simulink model "msdft_12_v2"  (R2013b)
settings: Solver=ode45  StartTime=0.0  StopTime=10.0  RelTol=1e-3
undefined symbols (not defined in the file or in its folder): msdft, sys_lib
libraries: xbsIndex_r4 x3195, casper_library_misc x152, casper_library_delays x42, dspsigops x32, xps_library x3
(part 10 of 33)

== system msdft_12_v2/msdft1/delay_tree4 ==
  in : Inport
  delay_c1_r1 : xbsIndex_r4/Delay  rst=off  infoeditControl=Selection of Reset will increase slice count due to use of real FFs and instead of SRLs  en=off  latency=1  dbl_ovrd=off  reg_retiming=on  block_type=delay
      settings: block_version=11.4
  delay_c2_r1 : xbsIndex_r4/Delay  rst=off  infoeditControl=Selection of Reset will increase slice count due to use of real FFs and instead of SRLs  en=off  latency=1  dbl_ovrd=off  reg_retiming=on  block_type=delay
      settings: block_version=11.4
  delay_c2_r2 : xbsIndex_r4/Delay  rst=off  infoeditControl=Selection of Reset will increase slice count due to use of real FFs and instead of SRLs  en=off  latency=1  dbl_ovrd=off  reg_retiming=on  block_type=delay
      settings: block_version=11.4
  delay_c3_r{1..4} (4 alike) : xbsIndex_r4/Delay  rst=off  infoeditControl=Selection of Reset will increase slice count due to use of real FFs and instead of SRLs  en=off  latency=1  dbl_ovrd=off  reg_retiming=on  block_type=delay
  delay_c4_r{1..8} (8 alike) : xbsIndex_r4/Delay  rst=off  infoeditControl=Selection of Reset will increase slice count due to use of real FFs and instead of SRLs  en=off  latency=1  dbl_ovrd=off  reg_retiming=on  block_type=delay
  term6 : Terminator
  term7 : Terminator
  term8 : Terminator
  out1 : Outport
  out2 : Outport  Port=2
  out3 : Outport  Port=3
  out4 : Outport  Port=4
  out5 : Outport  Port=5
  wires:
  in/1 -> delay_c1_r1/1
  delay_c1_r1/1 -> delay_c2_r1/1, delay_c2_r2/1
  delay_c2_r1/1 -> delay_c3_r1/1, delay_c3_r2/1
  delay_c2_r2/1 -> delay_c3_r3/1, delay_c3_r4/1
  delay_c3_r1/1 -> delay_c4_r1/1, delay_c4_r2/1
  delay_c3_r2/1 -> delay_c4_r3/1, delay_c4_r4/1
  delay_c3_r3/1 -> delay_c4_r5/1, delay_c4_r6/1
  delay_c3_r4/1 -> delay_c4_r7/1, delay_c4_r8/1
  delay_c4_r1/1 -> out1/1
  delay_c4_r2/1 -> out2/1
  delay_c4_r3/1 -> out3/1
  delay_c4_r4/1 -> out4/1
  delay_c4_r5/1 -> out5/1
  delay_c4_r6/1 -> term6/1
  delay_c4_r7/1 -> term7/1
  delay_c4_r8/1 -> term8/1

== system msdft_12_v2/msdft1/delay_tree5 ==
  in : Inport
  delay_c1_r1 : xbsIndex_r4/Delay  rst=off  infoeditControl=Selection of Reset will increase slice count due to use of real FFs and instead of SRLs  en=off  latency=1  dbl_ovrd=off  reg_retiming=on  block_type=delay
      settings: block_version=11.4
  delay_c2_r1 : xbsIndex_r4/Delay  rst=off  infoeditControl=Selection of Reset will increase slice count due to use of real FFs and instead of SRLs  en=off  latency=1  dbl_ovrd=off  reg_retiming=on  block_type=delay
      settings: block_version=11.4
  delay_c2_r2 : xbsIndex_r4/Delay  rst=off  infoeditControl=Selection of Reset will increase slice count due to use of real FFs and instead of SRLs  en=off  latency=1  dbl_ovrd=off  reg_retiming=on  block_type=delay
      settings: block_version=11.4
  delay_c3_r{1..4} (4 alike) : xbsIndex_r4/Delay  rst=off  infoeditControl=Selection of Reset will increase slice count due to use of real FFs and instead of SRLs  en=off  latency=1  dbl_ovrd=off  reg_retiming=on  block_type=delay
  delay_c4_r{1..8} (8 alike) : xbsIndex_r4/Delay  rst=off  infoeditControl=Selection of Reset will increase slice count due to use of real FFs and instead of SRLs  en=off  latency=1  dbl_ovrd=off  reg_retiming=on  block_type=delay
  term6 : Terminator
  term7 : Terminator
  term8 : Terminator
  out1 : Outport
  out2 : Outport  Port=2
  out3 : Outport  Port=3
  out4 : Outport  Port=4
  out5 : Outport  Port=5
  wires:
  in/1 -> delay_c1_r1/1
  delay_c1_r1/1 -> delay_c2_r1/1, delay_c2_r2/1
  delay_c2_r1/1 -> delay_c3_r1/1, delay_c3_r2/1
  delay_c2_r2/1 -> delay_c3_r3/1, delay_c3_r4/1
  delay_c3_r1/1 -> delay_c4_r1/1, delay_c4_r2/1
  delay_c3_r2/1 -> delay_c4_r3/1, delay_c4_r4/1
  delay_c3_r3/1 -> delay_c4_r5/1, delay_c4_r6/1
  delay_c3_r4/1 -> delay_c4_r7/1, delay_c4_r8/1
  delay_c4_r1/1 -> out1/1
  delay_c4_r2/1 -> out2/1
  delay_c4_r3/1 -> out3/1
  delay_c4_r4/1 -> out4/1
  delay_c4_r5/1 -> out5/1
  delay_c4_r6/1 -> term6/1
  delay_c4_r7/1 -> term7/1
  delay_c4_r8/1 -> term8/1

== system msdft_12_v2/msdft1/delay_tree6 ==
  in : Inport
  delay_c1_r1 : xbsIndex_r4/Delay  rst=off  infoeditControl=Selection of Reset will increase slice count due to use of real FFs and instead of SRLs  en=off  latency=1  dbl_ovrd=off  reg_retiming=on  block_type=delay
      settings: block_version=11.4
  delay_c2_r1 : xbsIndex_r4/Delay  rst=off  infoeditControl=Selection of Reset will increase slice count due to use of real FFs and instead of SRLs  en=off  latency=1  dbl_ovrd=off  reg_retiming=on  block_type=delay
      settings: block_version=11.4
  delay_c2_r2 : xbsIndex_r4/Delay  rst=off  infoeditControl=Selection of Reset will increase slice count due to use of real FFs and instead of SRLs  en=off  latency=1  dbl_ovrd=off  reg_retiming=on  block_type=delay
      settings: block_version=11.4
  delay_c3_r{1..4} (4 alike) : xbsIndex_r4/Delay  rst=off  infoeditControl=Selection of Reset will increase slice count due to use of real FFs and instead of SRLs  en=off  latency=1  dbl_ovrd=off  reg_retiming=on  block_type=delay
  delay_c4_r{1..8} (8 alike) : xbsIndex_r4/Delay  rst=off  infoeditControl=Selection of Reset will increase slice count due to use of real FFs and instead of SRLs  en=off  latency=1  dbl_ovrd=off  reg_retiming=on  block_type=delay
  term6 : Terminator
  term7 : Terminator
  term8 : Terminator
  out1 : Outport
  out2 : Outport  Port=2
  out3 : Outport  Port=3
  out4 : Outport  Port=4
  out5 : Outport  Port=5
  wires:
  in/1 -> delay_c1_r1/1
  delay_c1_r1/1 -> delay_c2_r1/1, delay_c2_r2/1
  delay_c2_r1/1 -> delay_c3_r1/1, delay_c3_r2/1
  delay_c2_r2/1 -> delay_c3_r3/1, delay_c3_r4/1
  delay_c3_r1/1 -> delay_c4_r1/1, delay_c4_r2/1
  delay_c3_r2/1 -> delay_c4_r3/1, delay_c4_r4/1
  delay_c3_r3/1 -> delay_c4_r5/1, delay_c4_r6/1
  delay_c3_r4/1 -> delay_c4_r7/1, delay_c4_r8/1
  delay_c4_r1/1 -> out1/1
  delay_c4_r2/1 -> out2/1
  delay_c4_r3/1 -> out3/1
  delay_c4_r4/1 -> out4/1
  delay_c4_r5/1 -> out5/1
  delay_c4_r6/1 -> term6/1
  delay_c4_r7/1 -> term7/1
  delay_c4_r8/1 -> term8/1

== system msdft_12_v2/msdft1/msdft ==
  note: see if saturates
  note: zero before
      | sync
  din : Inport
  sync : Inport  Port=2
  rst : Inport  Port=3
  twidd_im : Inport  Port=4
  twidd_re : Inport  Port=5
  we_twidd : Inport  Port=6
  mem_addr : Inport  Port=7
  Constant : xbsIndex_r4/Constant  const=1  gui_display_data_type=Boolean  arith_type=Boolean  n_bits=16  bin_pt=14  preci_type=Single  exp_width=8  frac_width=24  explicit_period=on  period=1  equ=P=C  opselect=C  inp2=PCIN>>17  opr=+  inp1=P  carry=CIN  dbl_ovrd=off  block_type=constant
  Convert : xbsIndex_r4/Convert  gui_display_data_type=Fixed-point  arith_type="Signed  (2's comp)"  n_bits=32  bin_pt=30  float_type=Single  exp_bits=8  fraction_bits=24  quantization=Truncate  overflow=Wrap  en=off  latency=0  dbl_ovrd=off  pipeline=off  block_type=convert
      settings: block_version=11.4
  Convert1 : xbsIndex_r4/Convert  gui_display_data_type=Fixed-point  arith_type="Signed  (2's comp)"  n_bits=32  bin_pt=30  float_type=Single  exp_bits=8  fraction_bits=24  quantization=Truncate  overflow=Wrap  en=off  latency=0  dbl_ovrd=off  pipeline=off  block_type=convert
      settings: block_version=11.4
  Delay : xbsIndex_r4/Delay  rst=off  infoeditControl=Selection of Reset will increase slice count due to use of real FFs and instead of SRLs  en=off  latency=5  dbl_ovrd=off  reg_retiming=off  block_type=delay
  Reinterpret : xbsIndex_r4/Reinterpret  force_arith_type=off  arith_type=Unsigned  force_bin_pt=on  bin_pt=twidd_bit-2  block_type=reinterpret
  Reinterpret1 : xbsIndex_r4/Reinterpret  force_arith_type=off  arith_type=Unsigned  force_bin_pt=on  bin_pt=twidd_bit-2  block_type=reinterpret
  Terminator : Terminator
  c_to_ri : casper_library_misc/c_to_ri  n_bits=16  bin_pt=14
      settings: AttributesFormatString=16_14 r/i
  cmult : Subsystem  AncestorBlock=casper_library_multipliers/cmult  mask(cmult){n_bits_a=in_bit+1, bin_pt_a=in_bit-1, n_bits_b=twidd_bit, bin_pt_b=twidd_bit-2, n_bits_ab=out_bit-N, bin_pt_ab=out_bit-N-5, quantization=Round  (unbiased: Even Values), overflow=Wrap, in_latency=0, mult_latency=3, add_latency=1, conv_latency=1, conjugated=off, async=off, pipelined_enable=on, multiplier_implementation=behavioral HDL}
      mask prompts: n_bits_a "Number of Bits 'a'"; bin_pt_a "Binary Point 'a'"; n_bits_b "Number of Bits 'b'"; bin_pt_b "Binary Point 'b'"; n_bits_ab "Number of Bits 'ab'"; bin_pt_ab "Binary Point 'ab'"; in_latency "Input latency"; mult_latency "Multiplier Latency"; add_latency "Adder Latency"; conv_latency "Convert latency"; conjugated "Conjugate"; async "asynchronous operation"; pipelined_enable "enable pipeline"; multiplier_implementation "Multiplier implementation"
      mask help:
      | Multiplies two complex numbers using 4 multipliers and 2 adders.
      | Conjugation is optional.
      mask init: same as msdft_12_v2/corrs/Subsystem/cmult
      settings: AttributesFormatString=|
      | 9_7 * 16_14 ==> 13_8
      | Round  (unbiased: Even Values), Wrap
      | Latency=0
      mask TypeOptions quantization: Truncate | Round  (unbiased: +/- Inf) | Round  (unbiased: Even Values)
      mask TypeOptions overflow: Wrap | Saturate | Flag as error
      mask TypeOptions multiplier_implementation: behavioral HDL | standard core | embedded multiplier core
  comb_filter : Subsystem  mask{N=N, bitwidth=in_bit}
      mask prompts: N "fft length (2^N)"
  done : Subsystem  Tag=xps:sw_reg  AncestorBlock=xps_library/software_register  mask(swreg){io_dir=To Processor, io_delay=0, sample_period=1, names=reg, bitwidths=32, bin_pts=0, arith_types=2, sim_port=on, show_format=on}
      mask prompts: io_dir "I/O direction"; io_delay "I/O delay"; sample_period "Sample period"; names "Bitfield names [msb...lsb]"; bitwidths "Bitfield widths"; bin_pts "Bitfield binary pts"; arith_types "Bitfield types, ufix=0, fix=1, bool=2"; sim_port "Provide sim input/output?"; show_format "Print format string?"
      mask help: A 32-bit software-accessible register. Can be divided into bitfields of varying widths and types using the fields in the block mask.
      mask init:
      | try
      |     swreg_init(gcb)
      | catch ex
      |     disp(sprintf('%s: %s', gcb, ex.message))
      |     errordlg(ex.message)
      | end
      settings: AttributesFormatString=1output:b = 32 bits
      mask TypeOptions io_dir: To Processor | From Processor
      mask Callback io_dir:
      | mask_enables = get_param(gcb, 'MaskEnables');
      | mask_names = get_param(gcb, 'MaskNames');
      | if strcmp(get_param(gcb, 'io_dir'), 'To Processor'),
      |     mask_enables{ismember(mask_names, 'sample_period')} = 'off';
      | else
      |     mask_enables{ismember(mask_names, 'sample_period')} = 'on';
      | end
      | set_param(gcb, 'MaskEnables', mask_enables);
  freeze_cntr : casper_library_misc/freeze_cntr  CounterBits=12
  pulse_ext : casper_library_misc/pulse_ext  pulse_len=2^8
  resonator : Subsystem  mask{in_bitwidth=out_bit-N, in_point=out_bit-N-5, N=N}
      mask prompts: in_bitwidth "input bitwidth"; in_point "input point"; N "fft length (2^?)"
  ri_to_c : casper_library_misc/ri_to_c
  rst_bram : Subsystem  Tag=xps:sw_reg  AncestorBlock=xps_library/software_register  mask(swreg){io_dir=From Processor, io_delay=0, sample_period=1, names=reg, bitwidths=32, bin_pts=0, arith_types=2, sim_port=on, show_format=on}
      mask prompts: io_dir "I/O direction"; io_delay "I/O delay"; sample_period "Sample period"; names "Bitfield names [msb...lsb]"; bitwidths "Bitfield widths"; bin_pts "Bitfield binary pts"; arith_types "Bitfield types, ufix=0, fix=1, bool=2"; sim_port "Provide sim input/output?"; show_format "Print format string?"
      mask help: A 32-bit software-accessible register. Can be divided into bitfields of varying widths and types using the fields in the block mask.
      mask init:
      | try
      |     swreg_init(gcb)
      | catch ex
      |     disp(sprintf('%s: %s', gcb, ex.message))
      |     errordlg(ex.message)
      | end
      settings: AttributesFormatString=1input:b = 32 bits
      mask TypeOptions io_dir: To Processor | From Processor
      mask Callback io_dir:
      | mask_enables = get_param(gcb, 'MaskEnables');
      | mask_names = get_param(gcb, 'MaskNames');
      | if strcmp(get_param(gcb, 'io_dir'), 'To Processor'),
      |     mask_enables{ismember(mask_names, 'sample_period')} = 'off';
      | else
      |     mask_enables{ismember(mask_names, 'sample_period')} = 'on';
      | end
      | set_param(gcb, 'MaskEnables', mask_enables);
  snapshot : Subsystem  Tag=casper:snapshot  AncestorBlock=casper_library_scopes/snapshot  mask(snapshot){storage=bram, dram_dimm=1, dram_clock=200, nsamples=10, data_width=64, offset=off, circap=off, value=off, use_dsp48=on}
      mask prompts: storage "Storage medium"; dram_dimm "DRAM dimm"; dram_clock "DRAM clock rate"; nsamples "Number of Samples (2^?)"; data_width "Data width"; offset "Start delay support"; circap "Circular capture support"; value "Extra value capture support"; use_dsp48 "Use DSP48s to implement counters"
      mask help:
      | Standard snap block, but with the following optional extras;
      |  1) Optionally delay the fabric trigger by a user-specified number of valids.
      |  2) Capture continuously after a trigger until a stop pulse is received. Data is captured into BRAM continuously, with old data being overwritten until a stop command is received. Then stop capturing when memory is filled. This enables you to get some data before and some data after the stop pulse. Use the 'tr_en_cnt' register to determine where you are in your vector. 'Addr' register's MSb now indicates 'busy capturing'.
      |  3) Optionally capture a value on an input port to a register at the same time as the first data sample.
      |  4) Implement counters using DSP48Es to save resources.
      mask init: same as msdft_12_v2/snapshot
      mask TypeOptions storage: bram | dram
      mask Callback storage: snapshot_callback();
      mask TypeOptions dram_dimm: 1 | 2 | 3 | 4
      mask TypeOptions dram_clock: 200 | 250 | 266 | 300 | 333
      mask TypeOptions data_width: 8 | 16 | 32 | 64 | 128
  twiddle_factor : Subsystem  mask{N=N, k=init_twidd, bitsize=twidd_bit}
      mask prompts: N "length FFT(2^)"; k "twiddle factor"; bitsize "bit size"
      mask help: RAM memories containing the twiddle adequate twiddle factors
  twidds : Subsystem  Tag=xps:bram  AncestorBlock=xps_library/Shared_BRAM  mask{arith_type=Unsigned, addr_width=12, data_width=64, reg_prim_output=off, reg_core_output=off, optimization=Minimum_Area, data_bin_pt=0, init_vals=[0:2^10-1], sample_rate=1}
      mask prompts: arith_type "Output Data Type"; addr_width "Address width"; data_width "Data Width"; reg_prim_output "Register Primitive Output"; reg_core_output "Register Core Output"; data_bin_pt "Data Binary Point"; init_vals "Initial values (simulation only)"; sample_rate "Sample rate"
      mask init:
      | shared_bram_mask;
      mask TypeOptions arith_type: Unsigned | Signed  (2's comp)
      mask TypeOptions data_width: 8 | 16 | 32 | 64 | 128
      mask TypeOptions optimization: Minimum_Area | Low_Power
  dout : Outport
  wires:
  Reinterpret1/1 -> twiddle_factor/6(im_data)
  Reinterpret/1 -> twiddle_factor/5(re_data)
  we_twidd/1 -> twiddle_factor/4(we_mem)
  sync/1 -> comb_filter/3(sync)
  [rst] -> comb_filter/2(rst)
  rst/1 -> [rst]
  comb_filter/1(dout) -> cmult/1(a)
  [rst] -> resonator/3(rst)
  Delay/1 -> resonator/2(sync)
  cmult/1(ab) -> resonator/1(din)
  twiddle_factor/2(sync_out) -> pulse_ext/1, Delay/1
  twiddle_factor/1(dout) -> cmult/2(b), c_to_ri/1
  twidd_im/1 -> Reinterpret1/1
  twidd_re/1 -> Reinterpret/1
  mem_addr/1 -> twiddle_factor/3(dir_mem)
  [rst] -> twiddle_factor/1(rst)
  comb_filter/2(sync_out) -> twiddle_factor/2(sync)
  resonator/1(dout) -> dout/1
  din/1 -> comb_filter/1(din)
  c_to_ri/1 -> Convert/1
  c_to_ri/2 -> Convert1/1
  Convert/1 -> ri_to_c/1
  Convert1/1 -> ri_to_c/2
  freeze_cntr/2 -> twidds/3(we)
  ri_to_c/1 -> snapshot/1(din), twidds/2(data_in)
  freeze_cntr/1 -> twidds/1(addr)
  pulse_ext/1 -> freeze_cntr/1
  rst_bram/1(in_reg) -> freeze_cntr/2
  freeze_cntr/3 -> done/1(out_reg)
  twidds/1(data_out) -> Terminator/1
  Constant/1 -> snapshot/2(we), snapshot/3(trig)

== system msdft_12_v2/msdft1/msdft1 ==
  note: see if saturates
  note: zero before
      | sync
  din : Inport
  sync : Inport  Port=2
  rst : Inport  Port=3
  twidd_im : Inport  Port=4
  twidd_re : Inport  Port=5
  we_twidd : Inport  Port=6
  mem_addr : Inport  Port=7
  Delay : xbsIndex_r4/Delay  rst=off  infoeditControl=Selection of Reset will increase slice count due to use of real FFs and instead of SRLs  en=off  latency=5  dbl_ovrd=off  reg_retiming=off  block_type=delay
  Reinterpret : xbsIndex_r4/Reinterpret  force_arith_type=off  arith_type=Unsigned  force_bin_pt=on  bin_pt=twidd_bit-2  block_type=reinterpret
  Reinterpret1 : xbsIndex_r4/Reinterpret  force_arith_type=off  arith_type=Unsigned  force_bin_pt=on  bin_pt=twidd_bit-2  block_type=reinterpret
  cmult : Subsystem  AncestorBlock=casper_library_multipliers/cmult  mask(cmult){n_bits_a=in_bit+1, bin_pt_a=in_bit-1, n_bits_b=twidd_bit, bin_pt_b=twidd_bit-2, n_bits_ab=out_bit-N, bin_pt_ab=out_bit-N-5, quantization=Round  (unbiased: Even Values), overflow=Wrap, in_latency=0, mult_latency=3, add_latency=1, conv_latency=1, conjugated=off, async=off, pipelined_enable=on, multiplier_implementation=behavioral HDL}
      mask prompts: n_bits_a "Number of Bits 'a'"; bin_pt_a "Binary Point 'a'"; n_bits_b "Number of Bits 'b'"; bin_pt_b "Binary Point 'b'"; n_bits_ab "Number of Bits 'ab'"; bin_pt_ab "Binary Point 'ab'"; in_latency "Input latency"; mult_latency "Multiplier Latency"; add_latency "Adder Latency"; conv_latency "Convert latency"; conjugated "Conjugate"; async "asynchronous operation"; pipelined_enable "enable pipeline"; multiplier_implementation "Multiplier implementation"
      mask help:
      | Multiplies two complex numbers using 4 multipliers and 2 adders.
      | Conjugation is optional.
      mask init: same as msdft_12_v2/corrs/Subsystem/cmult
      settings: AttributesFormatString=|
      | 9_7 * 16_14 ==> 13_8
      | Round  (unbiased: Even Values), Wrap
      | Latency=0
      mask TypeOptions quantization: Truncate | Round  (unbiased: +/- Inf) | Round  (unbiased: Even Values)
      mask TypeOptions overflow: Wrap | Saturate | Flag as error
      mask TypeOptions multiplier_implementation: behavioral HDL | standard core | embedded multiplier core
  comb_filter : Subsystem  mask{N=N, bitwidth=in_bit}
      mask prompts: N "fft length (2^N)"
  resonator : Subsystem  mask{in_bitwidth=out_bit-N, in_point=out_bit-N-5, N=N}
      mask prompts: in_bitwidth "input bitwidth"; in_point "input point"; N "fft length (2^?)"
  twiddle_factor : Subsystem  mask{N=N, k=init_twidd, bitsize=twidd_bit}
      mask prompts: N "length FFT(2^)"; k "twiddle factor"; bitsize "bit size"
      mask help: RAM memories containing the twiddle adequate twiddle factors
  dout : Outport
  wires:
  Reinterpret1/1 -> twiddle_factor/6(im_data)
  Reinterpret/1 -> twiddle_factor/5(re_data)
  we_twidd/1 -> twiddle_factor/4(we_mem)
  sync/1 -> comb_filter/3(sync)
  [rst] -> comb_filter/2(rst)
  rst/1 -> [rst]
  comb_filter/1(dout) -> cmult/1(a)
  [rst] -> resonator/3(rst)
  Delay/1 -> resonator/2(sync)
  cmult/1(ab) -> resonator/1(din)
  twiddle_factor/2(sync_out) -> Delay/1
  twiddle_factor/1(dout) -> cmult/2(b)
  twidd_im/1 -> Reinterpret1/1
  twidd_re/1 -> Reinterpret/1
  mem_addr/1 -> twiddle_factor/3(dir_mem)
  [rst] -> twiddle_factor/1(rst)
  comb_filter/2(sync_out) -> twiddle_factor/2(sync)
  resonator/1(dout) -> dout/1
  din/1 -> comb_filter/1(din)

== system msdft_12_v2/msdft1/msdft2 ==
  note: see if saturates
  note: zero before
      | sync
  din : Inport
  sync : Inport  Port=2
  rst : Inport  Port=3
  twidd_im : Inport  Port=4
  twidd_re : Inport  Port=5
  we_twidd : Inport  Port=6
  mem_addr : Inport  Port=7
  Delay : xbsIndex_r4/Delay  rst=off  infoeditControl=Selection of Reset will increase slice count due to use of real FFs and instead of SRLs  en=off  latency=5  dbl_ovrd=off  reg_retiming=off  block_type=delay
  Reinterpret : xbsIndex_r4/Reinterpret  force_arith_type=off  arith_type=Unsigned  force_bin_pt=on  bin_pt=twidd_bit-2  block_type=reinterpret
  Reinterpret1 : xbsIndex_r4/Reinterpret  force_arith_type=off  arith_type=Unsigned  force_bin_pt=on  bin_pt=twidd_bit-2  block_type=reinterpret
  cmult : Subsystem  AncestorBlock=casper_library_multipliers/cmult  mask(cmult){n_bits_a=in_bit+1, bin_pt_a=in_bit-1, n_bits_b=twidd_bit, bin_pt_b=twidd_bit-2, n_bits_ab=out_bit-N, bin_pt_ab=out_bit-N-5, quantization=Round  (unbiased: Even Values), overflow=Wrap, in_latency=0, mult_latency=3, add_latency=1, conv_latency=1, conjugated=off, async=off, pipelined_enable=on, multiplier_implementation=behavioral HDL}
      mask prompts: n_bits_a "Number of Bits 'a'"; bin_pt_a "Binary Point 'a'"; n_bits_b "Number of Bits 'b'"; bin_pt_b "Binary Point 'b'"; n_bits_ab "Number of Bits 'ab'"; bin_pt_ab "Binary Point 'ab'"; in_latency "Input latency"; mult_latency "Multiplier Latency"; add_latency "Adder Latency"; conv_latency "Convert latency"; conjugated "Conjugate"; async "asynchronous operation"; pipelined_enable "enable pipeline"; multiplier_implementation "Multiplier implementation"
      mask help:
      | Multiplies two complex numbers using 4 multipliers and 2 adders.
      | Conjugation is optional.
      mask init: same as msdft_12_v2/corrs/Subsystem/cmult
      settings: AttributesFormatString=|
      | 9_7 * 16_14 ==> 13_8
      | Round  (unbiased: Even Values), Wrap
      | Latency=0
      mask TypeOptions quantization: Truncate | Round  (unbiased: +/- Inf) | Round  (unbiased: Even Values)
      mask TypeOptions overflow: Wrap | Saturate | Flag as error
      mask TypeOptions multiplier_implementation: behavioral HDL | standard core | embedded multiplier core
  comb_filter : Subsystem  mask{N=N, bitwidth=in_bit}
      mask prompts: N "fft length (2^N)"
  resonator : Subsystem  mask{in_bitwidth=out_bit-N, in_point=out_bit-N-5, N=N}
      mask prompts: in_bitwidth "input bitwidth"; in_point "input point"; N "fft length (2^?)"
  twiddle_factor : Subsystem  mask{N=N, k=init_twidd, bitsize=twidd_bit}
      mask prompts: N "length FFT(2^)"; k "twiddle factor"; bitsize "bit size"
      mask help: RAM memories containing the twiddle adequate twiddle factors
  dout : Outport
  wires:
  Reinterpret1/1 -> twiddle_factor/6(im_data)
  Reinterpret/1 -> twiddle_factor/5(re_data)
  we_twidd/1 -> twiddle_factor/4(we_mem)
  sync/1 -> comb_filter/3(sync)
  [rst] -> comb_filter/2(rst)
  rst/1 -> [rst]
  comb_filter/1(dout) -> cmult/1(a)
  [rst] -> resonator/3(rst)
  Delay/1 -> resonator/2(sync)
  cmult/1(ab) -> resonator/1(din)
  twiddle_factor/2(sync_out) -> Delay/1
  twiddle_factor/1(dout) -> cmult/2(b)
  twidd_im/1 -> Reinterpret1/1
  twidd_re/1 -> Reinterpret/1
  mem_addr/1 -> twiddle_factor/3(dir_mem)
  [rst] -> twiddle_factor/1(rst)
  comb_filter/2(sync_out) -> twiddle_factor/2(sync)
  resonator/1(dout) -> dout/1
  din/1 -> comb_filter/1(din)

== system msdft_12_v2/msdft1/msdft3 ==
  note: see if saturates
  note: zero before
      | sync
  din : Inport
  sync : Inport  Port=2
  rst : Inport  Port=3
  twidd_im : Inport  Port=4
  twidd_re : Inport  Port=5
  we_twidd : Inport  Port=6
  mem_addr : Inport  Port=7
  Delay : xbsIndex_r4/Delay  rst=off  infoeditControl=Selection of Reset will increase slice count due to use of real FFs and instead of SRLs  en=off  latency=5  dbl_ovrd=off  reg_retiming=off  block_type=delay
  Reinterpret : xbsIndex_r4/Reinterpret  force_arith_type=off  arith_type=Unsigned  force_bin_pt=on  bin_pt=twidd_bit-2  block_type=reinterpret
  Reinterpret1 : xbsIndex_r4/Reinterpret  force_arith_type=off  arith_type=Unsigned  force_bin_pt=on  bin_pt=twidd_bit-2  block_type=reinterpret
  cmult : Subsystem  AncestorBlock=casper_library_multipliers/cmult  mask(cmult){n_bits_a=in_bit+1, bin_pt_a=in_bit-1, n_bits_b=twidd_bit, bin_pt_b=twidd_bit-2, n_bits_ab=out_bit-N, bin_pt_ab=out_bit-N-5, quantization=Round  (unbiased: Even Values), overflow=Wrap, in_latency=0, mult_latency=3, add_latency=1, conv_latency=1, conjugated=off, async=off, pipelined_enable=on, multiplier_implementation=behavioral HDL}
      mask prompts: n_bits_a "Number of Bits 'a'"; bin_pt_a "Binary Point 'a'"; n_bits_b "Number of Bits 'b'"; bin_pt_b "Binary Point 'b'"; n_bits_ab "Number of Bits 'ab'"; bin_pt_ab "Binary Point 'ab'"; in_latency "Input latency"; mult_latency "Multiplier Latency"; add_latency "Adder Latency"; conv_latency "Convert latency"; conjugated "Conjugate"; async "asynchronous operation"; pipelined_enable "enable pipeline"; multiplier_implementation "Multiplier implementation"
      mask help:
      | Multiplies two complex numbers using 4 multipliers and 2 adders.
      | Conjugation is optional.
      mask init: same as msdft_12_v2/corrs/Subsystem/cmult
      settings: AttributesFormatString=|
      | 9_7 * 16_14 ==> 13_8
      | Round  (unbiased: Even Values), Wrap
      | Latency=0
      mask TypeOptions quantization: Truncate | Round  (unbiased: +/- Inf) | Round  (unbiased: Even Values)
      mask TypeOptions overflow: Wrap | Saturate | Flag as error
      mask TypeOptions multiplier_implementation: behavioral HDL | standard core | embedded multiplier core
  comb_filter : Subsystem  mask{N=N, bitwidth=in_bit}
      mask prompts: N "fft length (2^N)"
  resonator : Subsystem  mask{in_bitwidth=out_bit-N, in_point=out_bit-N-5, N=N}
      mask prompts: in_bitwidth "input bitwidth"; in_point "input point"; N "fft length (2^?)"
  twiddle_factor : Subsystem  mask{N=N, k=init_twidd, bitsize=twidd_bit}
      mask prompts: N "length FFT(2^)"; k "twiddle factor"; bitsize "bit size"
      mask help: RAM memories containing the twiddle adequate twiddle factors
  dout : Outport
  wires:
  Reinterpret1/1 -> twiddle_factor/6(im_data)
  Reinterpret/1 -> twiddle_factor/5(re_data)
  we_twidd/1 -> twiddle_factor/4(we_mem)
  sync/1 -> comb_filter/3(sync)
  [rst] -> comb_filter/2(rst)
  rst/1 -> [rst]
  comb_filter/1(dout) -> cmult/1(a)
  [rst] -> resonator/3(rst)
  Delay/1 -> resonator/2(sync)
  cmult/1(ab) -> resonator/1(din)
  twiddle_factor/2(sync_out) -> Delay/1
  twiddle_factor/1(dout) -> cmult/2(b)
  twidd_im/1 -> Reinterpret1/1
  twidd_re/1 -> Reinterpret/1
  mem_addr/1 -> twiddle_factor/3(dir_mem)
  [rst] -> twiddle_factor/1(rst)
  comb_filter/2(sync_out) -> twiddle_factor/2(sync)
  resonator/1(dout) -> dout/1
  din/1 -> comb_filter/1(din)

== system msdft_12_v2/msdft1/msdft4 ==
  note: see if saturates
  note: zero before
      | sync
  din : Inport
  sync : Inport  Port=2
  rst : Inport  Port=3
  twidd_im : Inport  Port=4
  twidd_re : Inport  Port=5
  we_twidd : Inport  Port=6
  mem_addr : Inport  Port=7
  Delay : xbsIndex_r4/Delay  rst=off  infoeditControl=Selection of Reset will increase slice count due to use of real FFs and instead of SRLs  en=off  latency=5  dbl_ovrd=off  reg_retiming=off  block_type=delay
  Reinterpret : xbsIndex_r4/Reinterpret  force_arith_type=off  arith_type=Unsigned  force_bin_pt=on  bin_pt=twidd_bit-2  block_type=reinterpret
  Reinterpret1 : xbsIndex_r4/Reinterpret  force_arith_type=off  arith_type=Unsigned  force_bin_pt=on  bin_pt=twidd_bit-2  block_type=reinterpret
  cmult : Subsystem  AncestorBlock=casper_library_multipliers/cmult  mask(cmult){n_bits_a=in_bit+1, bin_pt_a=in_bit-1, n_bits_b=twidd_bit, bin_pt_b=twidd_bit-2, n_bits_ab=out_bit-N, bin_pt_ab=out_bit-N-5, quantization=Round  (unbiased: Even Values), overflow=Wrap, in_latency=0, mult_latency=3, add_latency=1, conv_latency=1, conjugated=off, async=off, pipelined_enable=on, multiplier_implementation=behavioral HDL}
      mask prompts: n_bits_a "Number of Bits 'a'"; bin_pt_a "Binary Point 'a'"; n_bits_b "Number of Bits 'b'"; bin_pt_b "Binary Point 'b'"; n_bits_ab "Number of Bits 'ab'"; bin_pt_ab "Binary Point 'ab'"; in_latency "Input latency"; mult_latency "Multiplier Latency"; add_latency "Adder Latency"; conv_latency "Convert latency"; conjugated "Conjugate"; async "asynchronous operation"; pipelined_enable "enable pipeline"; multiplier_implementation "Multiplier implementation"
      mask help:
      | Multiplies two complex numbers using 4 multipliers and 2 adders.
      | Conjugation is optional.
      mask init: same as msdft_12_v2/corrs/Subsystem/cmult
      settings: AttributesFormatString=|
      | 9_7 * 16_14 ==> 13_8
      | Round  (unbiased: Even Values), Wrap
      | Latency=0
      mask TypeOptions quantization: Truncate | Round  (unbiased: +/- Inf) | Round  (unbiased: Even Values)
      mask TypeOptions overflow: Wrap | Saturate | Flag as error
      mask TypeOptions multiplier_implementation: behavioral HDL | standard core | embedded multiplier core
  comb_filter : Subsystem  mask{N=N, bitwidth=in_bit}
      mask prompts: N "fft length (2^N)"
  resonator : Subsystem  mask{in_bitwidth=out_bit-N, in_point=out_bit-N-5, N=N}
      mask prompts: in_bitwidth "input bitwidth"; in_point "input point"; N "fft length (2^?)"
  twiddle_factor : Subsystem  mask{N=N, k=init_twidd, bitsize=twidd_bit}
      mask prompts: N "length FFT(2^)"; k "twiddle factor"; bitsize "bit size"
      mask help: RAM memories containing the twiddle adequate twiddle factors
  dout : Outport
  wires:
  Reinterpret1/1 -> twiddle_factor/6(im_data)
  Reinterpret/1 -> twiddle_factor/5(re_data)
  we_twidd/1 -> twiddle_factor/4(we_mem)
  sync/1 -> comb_filter/3(sync)
  [rst] -> comb_filter/2(rst)
  rst/1 -> [rst]
  comb_filter/1(dout) -> cmult/1(a)
  [rst] -> resonator/3(rst)
  Delay/1 -> resonator/2(sync)
  cmult/1(ab) -> resonator/1(din)
  twiddle_factor/2(sync_out) -> Delay/1
  twiddle_factor/1(dout) -> cmult/2(b)
  twidd_im/1 -> Reinterpret1/1
  twidd_re/1 -> Reinterpret/1
  mem_addr/1 -> twiddle_factor/3(dir_mem)
  [rst] -> twiddle_factor/1(rst)
  comb_filter/2(sync_out) -> twiddle_factor/2(sync)
  resonator/1(dout) -> dout/1
  din/1 -> comb_filter/1(din)

== system msdft_12_v2/msdft2/delay_tree ==
  in : Inport
  delay_c1_r1 : xbsIndex_r4/Delay  rst=off  infoeditControl=Selection of Reset will increase slice count due to use of real FFs and instead of SRLs  en=off  latency=1  dbl_ovrd=off  reg_retiming=on  block_type=delay
      settings: block_version=11.4
  delay_c2_r1 : xbsIndex_r4/Delay  rst=off  infoeditControl=Selection of Reset will increase slice count due to use of real FFs and instead of SRLs  en=off  latency=1  dbl_ovrd=off  reg_retiming=on  block_type=delay
      settings: block_version=11.4
  delay_c2_r2 : xbsIndex_r4/Delay  rst=off  infoeditControl=Selection of Reset will increase slice count due to use of real FFs and instead of SRLs  en=off  latency=1  dbl_ovrd=off  reg_retiming=on  block_type=delay
      settings: block_version=11.4
  delay_c3_r{1..4} (4 alike) : xbsIndex_r4/Delay  rst=off  infoeditControl=Selection of Reset will increase slice count due to use of real FFs and instead of SRLs  en=off  latency=1  dbl_ovrd=off  reg_retiming=on  block_type=delay
  delay_c4_r{1..8} (8 alike) : xbsIndex_r4/Delay  rst=off  infoeditControl=Selection of Reset will increase slice count due to use of real FFs and instead of SRLs  en=off  latency=1  dbl_ovrd=off  reg_retiming=on  block_type=delay
  term6 : Terminator
  term7 : Terminator
  term8 : Terminator
  out1 : Outport
  out2 : Outport  Port=2
  out3 : Outport  Port=3
  out4 : Outport  Port=4
  out5 : Outport  Port=5
  wires:
  in/1 -> delay_c1_r1/1
  delay_c1_r1/1 -> delay_c2_r1/1, delay_c2_r2/1
  delay_c2_r1/1 -> delay_c3_r1/1, delay_c3_r2/1
  delay_c2_r2/1 -> delay_c3_r3/1, delay_c3_r4/1
  delay_c3_r1/1 -> delay_c4_r1/1, delay_c4_r2/1
  delay_c3_r2/1 -> delay_c4_r3/1, delay_c4_r4/1
  delay_c3_r3/1 -> delay_c4_r5/1, delay_c4_r6/1
  delay_c3_r4/1 -> delay_c4_r7/1, delay_c4_r8/1
  delay_c4_r1/1 -> out1/1
  delay_c4_r2/1 -> out2/1
  delay_c4_r3/1 -> out3/1
  delay_c4_r4/1 -> out4/1
  delay_c4_r5/1 -> out5/1
  delay_c4_r6/1 -> term6/1
  delay_c4_r7/1 -> term7/1
  delay_c4_r8/1 -> term8/1

== system msdft_12_v2/msdft2/delay_tree1 ==
  in : Inport
  delay_c1_r1 : xbsIndex_r4/Delay  rst=off  infoeditControl=Selection of Reset will increase slice count due to use of real FFs and instead of SRLs  en=off  latency=1  dbl_ovrd=off  reg_retiming=on  block_type=delay
      settings: block_version=11.4
  delay_c2_r1 : xbsIndex_r4/Delay  rst=off  infoeditControl=Selection of Reset will increase slice count due to use of real FFs and instead of SRLs  en=off  latency=1  dbl_ovrd=off  reg_retiming=on  block_type=delay
      settings: block_version=11.4
  delay_c2_r2 : xbsIndex_r4/Delay  rst=off  infoeditControl=Selection of Reset will increase slice count due to use of real FFs and instead of SRLs  en=off  latency=1  dbl_ovrd=off  reg_retiming=on  block_type=delay
      settings: block_version=11.4
  delay_c3_r{1..4} (4 alike) : xbsIndex_r4/Delay  rst=off  infoeditControl=Selection of Reset will increase slice count due to use of real FFs and instead of SRLs  en=off  latency=1  dbl_ovrd=off  reg_retiming=on  block_type=delay
  delay_c4_r{1..8} (8 alike) : xbsIndex_r4/Delay  rst=off  infoeditControl=Selection of Reset will increase slice count due to use of real FFs and instead of SRLs  en=off  latency=1  dbl_ovrd=off  reg_retiming=on  block_type=delay
  term6 : Terminator
  term7 : Terminator
  term8 : Terminator
  out1 : Outport
  out2 : Outport  Port=2
  out3 : Outport  Port=3
  out4 : Outport  Port=4
  out5 : Outport  Port=5
  wires:
  in/1 -> delay_c1_r1/1
  delay_c1_r1/1 -> delay_c2_r1/1, delay_c2_r2/1
  delay_c2_r1/1 -> delay_c3_r1/1, delay_c3_r2/1
  delay_c2_r2/1 -> delay_c3_r3/1, delay_c3_r4/1
  delay_c3_r1/1 -> delay_c4_r1/1, delay_c4_r2/1
  delay_c3_r2/1 -> delay_c4_r3/1, delay_c4_r4/1
  delay_c3_r3/1 -> delay_c4_r5/1, delay_c4_r6/1
  delay_c3_r4/1 -> delay_c4_r7/1, delay_c4_r8/1
  delay_c4_r1/1 -> out1/1
  delay_c4_r2/1 -> out2/1
  delay_c4_r3/1 -> out3/1
  delay_c4_r4/1 -> out4/1
  delay_c4_r5/1 -> out5/1
  delay_c4_r6/1 -> term6/1
  delay_c4_r7/1 -> term7/1
  delay_c4_r8/1 -> term8/1

== system msdft_12_v2/msdft2/delay_tree2 ==
  in : Inport
  delay_c1_r1 : xbsIndex_r4/Delay  rst=off  infoeditControl=Selection of Reset will increase slice count due to use of real FFs and instead of SRLs  en=off  latency=1  dbl_ovrd=off  reg_retiming=on  block_type=delay
      settings: block_version=11.4
  delay_c2_r1 : xbsIndex_r4/Delay  rst=off  infoeditControl=Selection of Reset will increase slice count due to use of real FFs and instead of SRLs  en=off  latency=1  dbl_ovrd=off  reg_retiming=on  block_type=delay
      settings: block_version=11.4
  delay_c2_r2 : xbsIndex_r4/Delay  rst=off  infoeditControl=Selection of Reset will increase slice count due to use of real FFs and instead of SRLs  en=off  latency=1  dbl_ovrd=off  reg_retiming=on  block_type=delay
      settings: block_version=11.4
  delay_c3_r{1..4} (4 alike) : xbsIndex_r4/Delay  rst=off  infoeditControl=Selection of Reset will increase slice count due to use of real FFs and instead of SRLs  en=off  latency=1  dbl_ovrd=off  reg_retiming=on  block_type=delay
  delay_c4_r{1..8} (8 alike) : xbsIndex_r4/Delay  rst=off  infoeditControl=Selection of Reset will increase slice count due to use of real FFs and instead of SRLs  en=off  latency=1  dbl_ovrd=off  reg_retiming=on  block_type=delay
  term6 : Terminator
  term7 : Terminator
  term8 : Terminator
  out1 : Outport
  out2 : Outport  Port=2
  out3 : Outport  Port=3
  out4 : Outport  Port=4
  out5 : Outport  Port=5
  wires:
  in/1 -> delay_c1_r1/1
  delay_c1_r1/1 -> delay_c2_r1/1, delay_c2_r2/1
  delay_c2_r1/1 -> delay_c3_r1/1, delay_c3_r2/1
  delay_c2_r2/1 -> delay_c3_r3/1, delay_c3_r4/1
  delay_c3_r1/1 -> delay_c4_r1/1, delay_c4_r2/1
  delay_c3_r2/1 -> delay_c4_r3/1, delay_c4_r4/1
  delay_c3_r3/1 -> delay_c4_r5/1, delay_c4_r6/1
  delay_c3_r4/1 -> delay_c4_r7/1, delay_c4_r8/1
  delay_c4_r1/1 -> out1/1
  delay_c4_r2/1 -> out2/1
  delay_c4_r3/1 -> out3/1
  delay_c4_r4/1 -> out4/1
  delay_c4_r5/1 -> out5/1
  delay_c4_r6/1 -> term6/1
  delay_c4_r7/1 -> term7/1
  delay_c4_r8/1 -> term8/1

== system msdft_12_v2/msdft2/delay_tree3 ==
  in : Inport
  delay_c1_r1 : xbsIndex_r4/Delay  rst=off  infoeditControl=Selection of Reset will increase slice count due to use of real FFs and instead of SRLs  en=off  latency=1  dbl_ovrd=off  reg_retiming=on  block_type=delay
      settings: block_version=11.4
  delay_c2_r1 : xbsIndex_r4/Delay  rst=off  infoeditControl=Selection of Reset will increase slice count due to use of real FFs and instead of SRLs  en=off  latency=1  dbl_ovrd=off  reg_retiming=on  block_type=delay
      settings: block_version=11.4
  delay_c2_r2 : xbsIndex_r4/Delay  rst=off  infoeditControl=Selection of Reset will increase slice count due to use of real FFs and instead of SRLs  en=off  latency=1  dbl_ovrd=off  reg_retiming=on  block_type=delay
      settings: block_version=11.4
  delay_c3_r{1..4} (4 alike) : xbsIndex_r4/Delay  rst=off  infoeditControl=Selection of Reset will increase slice count due to use of real FFs and instead of SRLs  en=off  latency=1  dbl_ovrd=off  reg_retiming=on  block_type=delay
  delay_c4_r{1..8} (8 alike) : xbsIndex_r4/Delay  rst=off  infoeditControl=Selection of Reset will increase slice count due to use of real FFs and instead of SRLs  en=off  latency=1  dbl_ovrd=off  reg_retiming=on  block_type=delay
  term6 : Terminator
  term7 : Terminator
  term8 : Terminator
  out1 : Outport
  out2 : Outport  Port=2
  out3 : Outport  Port=3
  out4 : Outport  Port=4
  out5 : Outport  Port=5
  wires:
  in/1 -> delay_c1_r1/1
  delay_c1_r1/1 -> delay_c2_r1/1, delay_c2_r2/1
  delay_c2_r1/1 -> delay_c3_r1/1, delay_c3_r2/1
  delay_c2_r2/1 -> delay_c3_r3/1, delay_c3_r4/1
  delay_c3_r1/1 -> delay_c4_r1/1, delay_c4_r2/1
  delay_c3_r2/1 -> delay_c4_r3/1, delay_c4_r4/1
  delay_c3_r3/1 -> delay_c4_r5/1, delay_c4_r6/1
  delay_c3_r4/1 -> delay_c4_r7/1, delay_c4_r8/1
  delay_c4_r1/1 -> out1/1
  delay_c4_r2/1 -> out2/1
  delay_c4_r3/1 -> out3/1
  delay_c4_r4/1 -> out4/1
  delay_c4_r5/1 -> out5/1
  delay_c4_r6/1 -> term6/1
  delay_c4_r7/1 -> term7/1
  delay_c4_r8/1 -> term8/1

== system msdft_12_v2/msdft2/delay_tree4 ==
  in : Inport
  delay_c1_r1 : xbsIndex_r4/Delay  rst=off  infoeditControl=Selection of Reset will increase slice count due to use of real FFs and instead of SRLs  en=off  latency=1  dbl_ovrd=off  reg_retiming=on  block_type=delay
      settings: block_version=11.4
  delay_c2_r1 : xbsIndex_r4/Delay  rst=off  infoeditControl=Selection of Reset will increase slice count due to use of real FFs and instead of SRLs  en=off  latency=1  dbl_ovrd=off  reg_retiming=on  block_type=delay
      settings: block_version=11.4
  delay_c2_r2 : xbsIndex_r4/Delay  rst=off  infoeditControl=Selection of Reset will increase slice count due to use of real FFs and instead of SRLs  en=off  latency=1  dbl_ovrd=off  reg_retiming=on  block_type=delay
      settings: block_version=11.4
  delay_c3_r{1..4} (4 alike) : xbsIndex_r4/Delay  rst=off  infoeditControl=Selection of Reset will increase slice count due to use of real FFs and instead of SRLs  en=off  latency=1  dbl_ovrd=off  reg_retiming=on  block_type=delay
  delay_c4_r{1..8} (8 alike) : xbsIndex_r4/Delay  rst=off  infoeditControl=Selection of Reset will increase slice count due to use of real FFs and instead of SRLs  en=off  latency=1  dbl_ovrd=off  reg_retiming=on  block_type=delay
  term6 : Terminator
  term7 : Terminator
  term8 : Terminator
  out1 : Outport
  out2 : Outport  Port=2
  out3 : Outport  Port=3
  out4 : Outport  Port=4
  out5 : Outport  Port=5
  wires:
  in/1 -> delay_c1_r1/1
  delay_c1_r1/1 -> delay_c2_r1/1, delay_c2_r2/1
  delay_c2_r1/1 -> delay_c3_r1/1, delay_c3_r2/1
  delay_c2_r2/1 -> delay_c3_r3/1, delay_c3_r4/1
  delay_c3_r1/1 -> delay_c4_r1/1, delay_c4_r2/1
  delay_c3_r2/1 -> delay_c4_r3/1, delay_c4_r4/1
  delay_c3_r3/1 -> delay_c4_r5/1, delay_c4_r6/1
  delay_c3_r4/1 -> delay_c4_r7/1, delay_c4_r8/1
  delay_c4_r1/1 -> out1/1
  delay_c4_r2/1 -> out2/1
  delay_c4_r3/1 -> out3/1
  delay_c4_r4/1 -> out4/1
  delay_c4_r5/1 -> out5/1
  delay_c4_r6/1 -> term6/1
  delay_c4_r7/1 -> term7/1
  delay_c4_r8/1 -> term8/1

== system msdft_12_v2/msdft2/delay_tree5 ==
  in : Inport
  delay_c1_r1 : xbsIndex_r4/Delay  rst=off  infoeditControl=Selection of Reset will increase slice count due to use of real FFs and instead of SRLs  en=off  latency=1  dbl_ovrd=off  reg_retiming=on  block_type=delay
      settings: block_version=11.4
  delay_c2_r1 : xbsIndex_r4/Delay  rst=off  infoeditControl=Selection of Reset will increase slice count due to use of real FFs and instead of SRLs  en=off  latency=1  dbl_ovrd=off  reg_retiming=on  block_type=delay
      settings: block_version=11.4
  delay_c2_r2 : xbsIndex_r4/Delay  rst=off  infoeditControl=Selection of Reset will increase slice count due to use of real FFs and instead of SRLs  en=off  latency=1  dbl_ovrd=off  reg_retiming=on  block_type=delay
      settings: block_version=11.4
  delay_c3_r{1..4} (4 alike) : xbsIndex_r4/Delay  rst=off  infoeditControl=Selection of Reset will increase slice count due to use of real FFs and instead of SRLs  en=off  latency=1  dbl_ovrd=off  reg_retiming=on  block_type=delay
  delay_c4_r{1..8} (8 alike) : xbsIndex_r4/Delay  rst=off  infoeditControl=Selection of Reset will increase slice count due to use of real FFs and instead of SRLs  en=off  latency=1  dbl_ovrd=off  reg_retiming=on  block_type=delay
  term6 : Terminator
  term7 : Terminator
  term8 : Terminator
  out1 : Outport
  out2 : Outport  Port=2
  out3 : Outport  Port=3
  out4 : Outport  Port=4
  out5 : Outport  Port=5
  wires:
  in/1 -> delay_c1_r1/1
  delay_c1_r1/1 -> delay_c2_r1/1, delay_c2_r2/1
  delay_c2_r1/1 -> delay_c3_r1/1, delay_c3_r2/1
  delay_c2_r2/1 -> delay_c3_r3/1, delay_c3_r4/1
  delay_c3_r1/1 -> delay_c4_r1/1, delay_c4_r2/1
  delay_c3_r2/1 -> delay_c4_r3/1, delay_c4_r4/1
  delay_c3_r3/1 -> delay_c4_r5/1, delay_c4_r6/1
  delay_c3_r4/1 -> delay_c4_r7/1, delay_c4_r8/1
  delay_c4_r1/1 -> out1/1
  delay_c4_r2/1 -> out2/1
  delay_c4_r3/1 -> out3/1
  delay_c4_r4/1 -> out4/1
  delay_c4_r5/1 -> out5/1
  delay_c4_r6/1 -> term6/1
  delay_c4_r7/1 -> term7/1
  delay_c4_r8/1 -> term8/1

== system msdft_12_v2/msdft2/delay_tree6 ==
  in : Inport
  delay_c1_r1 : xbsIndex_r4/Delay  rst=off  infoeditControl=Selection of Reset will increase slice count due to use of real FFs and instead of SRLs  en=off  latency=1  dbl_ovrd=off  reg_retiming=on  block_type=delay
      settings: block_version=11.4
  delay_c2_r1 : xbsIndex_r4/Delay  rst=off  infoeditControl=Selection of Reset will increase slice count due to use of real FFs and instead of SRLs  en=off  latency=1  dbl_ovrd=off  reg_retiming=on  block_type=delay
      settings: block_version=11.4
  delay_c2_r2 : xbsIndex_r4/Delay  rst=off  infoeditControl=Selection of Reset will increase slice count due to use of real FFs and instead of SRLs  en=off  latency=1  dbl_ovrd=off  reg_retiming=on  block_type=delay
      settings: block_version=11.4
  delay_c3_r{1..4} (4 alike) : xbsIndex_r4/Delay  rst=off  infoeditControl=Selection of Reset will increase slice count due to use of real FFs and instead of SRLs  en=off  latency=1  dbl_ovrd=off  reg_retiming=on  block_type=delay
  delay_c4_r{1..8} (8 alike) : xbsIndex_r4/Delay  rst=off  infoeditControl=Selection of Reset will increase slice count due to use of real FFs and instead of SRLs  en=off  latency=1  dbl_ovrd=off  reg_retiming=on  block_type=delay
  term6 : Terminator
  term7 : Terminator
  term8 : Terminator
  out1 : Outport
  out2 : Outport  Port=2
  out3 : Outport  Port=3
  out4 : Outport  Port=4
  out5 : Outport  Port=5
  wires:
  in/1 -> delay_c1_r1/1
  delay_c1_r1/1 -> delay_c2_r1/1, delay_c2_r2/1
  delay_c2_r1/1 -> delay_c3_r1/1, delay_c3_r2/1
  delay_c2_r2/1 -> delay_c3_r3/1, delay_c3_r4/1
  delay_c3_r1/1 -> delay_c4_r1/1, delay_c4_r2/1
  delay_c3_r2/1 -> delay_c4_r3/1, delay_c4_r4/1
  delay_c3_r3/1 -> delay_c4_r5/1, delay_c4_r6/1
  delay_c3_r4/1 -> delay_c4_r7/1, delay_c4_r8/1
  delay_c4_r1/1 -> out1/1
  delay_c4_r2/1 -> out2/1
  delay_c4_r3/1 -> out3/1
  delay_c4_r4/1 -> out4/1
  delay_c4_r5/1 -> out5/1
  delay_c4_r6/1 -> term6/1
  delay_c4_r7/1 -> term7/1
  delay_c4_r8/1 -> term8/1
